simulink model "CSTR_Model"  (R2022b)
settings: Solver=ode15s  StartTime=0.0  StopTime=inf  RelTol=1e-3  EnableMultiTasking=on
InitFcn:
  | CSTR_Setup
undefined symbols (not defined in the file): CAf, Tf
libraries: jMPClib x3, simulink x1, vrlib x1
settings Model: Creator=Jonathan Currie  LastModifiedBy=Jonathan Currie
settings SolverCC: AlgebraicLoopSolver=TrustRegion
settings DataIOCC: LimitDataPoints=on  SaveFormat=Array  SignalLoggingSaveFormat=ModelDataLogs  ReturnWorkspaceOutputs=off
settings OptimizationCC: ExpressionDepthLimit=2147483647  LifeSpan=inf
settings DebuggingCC: UnderspecifiedInitializationDetection=Classic  MergeDetectMultiDrivingBlocksExec=none  SolverPrmCheckMsg=warning  FcnCallInpInsideContextMsg=warning  UnconnectedInputMsg=warning  UnconnectedOutputMsg=warning  UnconnectedLineMsg=warning  StateNameClashWarn=warning  SFUnexpectedBacktrackingDiag=warning  SFNoUnconditionalDefaultTransitionDiag=warning  SFExecutionAtInitializationDiag=none  SFMachineParentedDataDiag=warning  ArithmeticOperatorsInVariantConditions=warning
settings HardwareCC: ProdBitPerPointer=32  ProdBitPerSizeT=32  ProdBitPerPtrDiffT=32  ProdLargestAtomicFloat=None  ProdIntDivRoundTo=Undefined  ProdEndianess=Unspecified  ProdWordSize=32  ProdHWDeviceType=32-bit Generic
settings ModelReferenceCC: PropagateSignalLabelsOutOfModel=off
settings SFSimCC: SimUseLocalCustomCode=off  CustomCodeUndefinedFunction=UseInterfaceOnly
settings RTWCC: RTWUseLocalCustomCode=off
settings CodeAppCC: StateflowObjectComments=on
settings GRTTargetCC: TargetLangStandard=C89/C90 (ANSI)  CombineOutputUpdateFcns=off  GRTInterface=on
settings ConfigComp: CovMetricSettings=dw  CovSaveCumulativeToWorkspaceVar=on  CovSaveSingleToWorkspaceVar=on  CovExternalEMLEnable=off

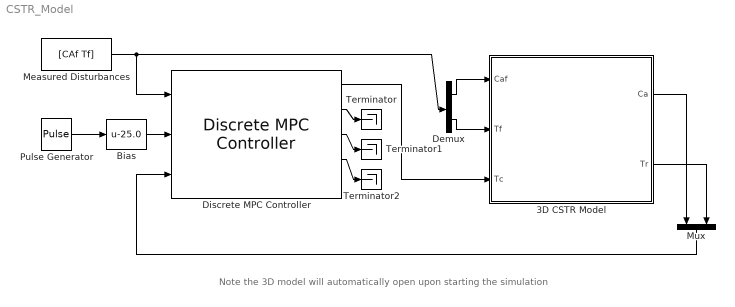
== system CSTR_Model ==
  note: Note the 3D model will automatically open upon starting the simulation
  3D CSTR Model : Subsystem
      mask Display:
      | image(imread('Images/CSTRblock.png'))
      | port_label('input', 1, 'Caf')
      | port_label('input', 2, 'Tf')
      | port_label('input', 3, 'Tc')
      | port_label('output', 1, 'Ca')
      | port_label('output', 2, 'Tr')
  Bias : Bias  Bias=-25.0  SaturateOnIntegerOverflow=off
  Demux : Demux  Outputs=2
  Discrete MPC Controller : jMPClib/MPC Blocks/Discrete MPC Controller  SIMJMPC=MPC1
      settings: SourceProductName=JMPC Toolbox
  Measured Disturbances : Constant  Value=[CAf Tf]
  Mux : Mux  Inputs=2
  Pulse Generator : DiscretePulseGenerator  PulseType=Time based  Amplitude=50  Period=20  PulseWidth=50
  Terminator : Terminator
  Terminator1 : Terminator
  Terminator2 : Terminator
  wires:
  Measured Disturbances/1 -> Discrete MPC Controller/1, Demux/1
  3D CSTR Model/1(Ca) -> Mux/1
  3D CSTR Model/2(Tr) -> Mux/2
  Mux/1 -> Discrete MPC Controller/3
  Demux/2 -> 3D CSTR Model/2(Tf)
  Demux/1 -> 3D CSTR Model/1(Caf)
  Pulse Generator/1 -> Bias/1
  Discrete MPC Controller/2 -> Terminator/1
  Discrete MPC Controller/3 -> Terminator1/1
  Discrete MPC Controller/4 -> Terminator2/1
  Bias/1 -> Discrete MPC Controller/2
  Discrete MPC Controller/1 -> 3D CSTR Model/3(Tc)

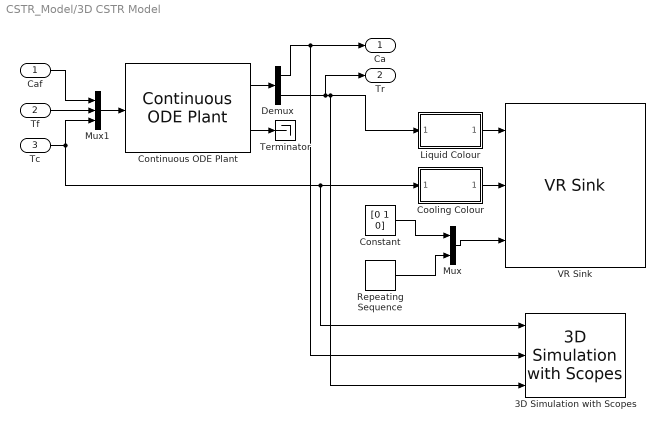
== system CSTR_Model/3D CSTR Model ==
  Caf : Inport
  Tf : Inport  Port=2
  Tc : Inport  Port=3
  3D Simulation with Scopes : jMPClib/Displays/3D Simulation with Scopes  vrw=vrw  titles=titles  limits=ylims  tlim=tlim  viden=0
      settings: SourceProductName=JMPC Toolbox
  Constant : Constant  Value=[0 1 0]
  Continuous ODE Plant : jMPClib/MPC Blocks/Continuous ODE Plant  jNLObj=Plant
      settings: SourceProductName=JMPC Toolbox
  Cooling Colour : Subsystem
  Demux : Demux  Outputs=2
  Liquid Colour : Subsystem
  Mux : Mux  Inputs=2
  Mux1 : Mux  Inputs=3
  Repeating Sequence : simulink/Sources/Repeating Sequence  rep_seq_t=0:30  rep_seq_y=linspace(0,20*pi,31)
  Terminator : Terminator
  VR Sink : vrlib/VR Sink  InstantiateOnLoad=on  SampleTime=0.1  ViewEnable=on  RemoteChange=off  RemoteView=on  FieldsWritten=LiqMat.diffuseColor.3.1.1.double#CoolMat.diffuseColor.3.1.1.double#Stirrer.rotation.4.1.1.double  WorldFileName=CSTR.wrl  WorldDescription=CSTR  AutoView=on  VideoDimensions=[]  AllowVariableSize=off  FigureProperties="{'Position', 'Name', 'Viewpoint', 'CameraBound', 'CameraDirection', 'CameraPosition', 'CameraUpVector', 'ZoomFactor', 'Antialiasing', 'Headlight', 'Lighting', 'NavPanel', 'Sound', 'StatusBar', 'Stereo3D', 'Stereo3DCameraOffset', 'Stereo3DHIT', 'ToolBar', 'Textures', 'Transparency', 'Triad', 'Wireframe', 'NavZones', 'NavMode', 'NavSpeed', 'CaptureFileFormat', 'CaptureFileName', 'Record2DCompressMethod', 'Record2DCompressQuality', 'Record2D', 'Record2DFileName', 'Record2DFPS'; [5.0000000000000000e+00   9.2000000000000000e+01   5.7600000000000000e+02   3.5000000000000000e+02], 'CSTR', 'Normal', 'on', [0.0000000000000000e+00   0.0000000000000000e+00  -1.0000000000000000e+00], [0.0000000000000000e+00   0.0000000000000000e+00   0.0000000000000000e+00], [0.0000000000000000e+00   1.0000000000000000e+00   0.0000000000000000e+00], [1.0000000000000000e+00], 'off', 'on', 'on', 'halfbar', 'on', 'on', 'off', [1.0000000149011612e-01], [0.0000000000000000e+00], 'on', 'on', 'on', 'none', 'off', 'off', 'fly', 'normal', 'tif', '%f_anim_%n.tif', 'auto', [7.5000000000000000e+01], 'off', '%f_anim_%n.avi', 'auto'}"
  Ca : Outport
  Tr : Outport  Port=2
  wires:
  Liquid Colour/1(LiqCol) -> VR Sink/1
  Cooling Colour/1(LiqCol) -> VR Sink/2
  Mux/1 -> VR Sink/3
  Constant/1 -> Mux/1
  Continuous ODE Plant/1 -> Demux/1
  Demux/2 -> Tr/1, Liquid Colour/1(Temp), 3D Simulation with Scopes/3
  Continuous ODE Plant/2 -> Terminator/1
  Demux/1 -> Ca/1, 3D Simulation with Scopes/2
  Tc/1 -> Mux1/3, Cooling Colour/1(Temp), 3D Simulation with Scopes/1
  Mux1/1 -> Continuous ODE Plant/1
  Tf/1 -> Mux1/2
  Caf/1 -> Mux1/1
  Repeating Sequence/1 -> Mux/2

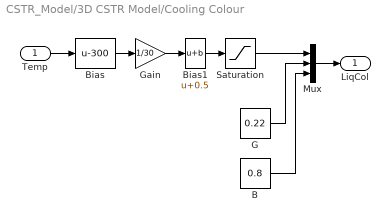
== system CSTR_Model/3D CSTR Model/Cooling Colour ==
  Temp : Inport
  B : Constant  Value=0.8
  Bias : Bias  Bias=-300  SaturateOnIntegerOverflow=off
  Bias1 : Bias  Bias=0.5  SaturateOnIntegerOverflow=off
  G : Constant  Value=0.22
  Gain : Gain  Gain=1/30
  Mux : Mux  Inputs=3
  Saturation : Saturate  UpperLimit=1  LowerLimit=0
  LiqCol : Outport
  wires:
  Mux/1 -> LiqCol/1
  Temp/1 -> Bias/1
  Bias1/1 -> Saturation/1
  Gain/1 -> Bias1/1
  Saturation/1 -> Mux/1
  Bias/1 -> Gain/1
  B/1 -> Mux/3
  G/1 -> Mux/2

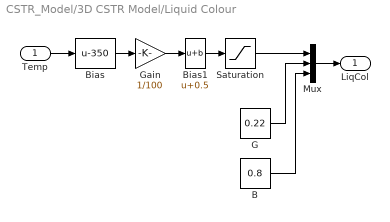
== system CSTR_Model/3D CSTR Model/Liquid Colour ==
  Temp : Inport
  B : Constant  Value=0.8
  Bias : Bias  Bias=-350  SaturateOnIntegerOverflow=off
  Bias1 : Bias  Bias=0.5  SaturateOnIntegerOverflow=off
  G : Constant  Value=0.22
  Gain : Gain  Gain=1/100
  Mux : Mux  Inputs=3
  Saturation : Saturate  UpperLimit=1  LowerLimit=0
  LiqCol : Outport
  wires:
  G/1 -> Mux/2
  B/1 -> Mux/3
  Bias/1 -> Gain/1
  Saturation/1 -> Mux/1
  Gain/1 -> Bias1/1
  Bias1/1 -> Saturation/1
  Temp/1 -> Bias/1
  Mux/1 -> LiqCol/1
